simulink model "MPPT_INC"  (R2018a)
settings: Solver=ode23s  StartTime=0.0  StopTime=1200  MaxStep=1e-5  RelTol=1e-4  EnableMultiTasking=on
libraries: powerlib x7, powerlib_meascontrol x1, re_lib x1, simulink x1
settings Model: Creator=HP  LastModifiedBy=yusuf
settings SolverCC: ZeroCrossControl=DisableAll  AlgebraicLoopSolver=LineSearch
settings DataIOCC: LimitDataPoints=on  SaveFormat=Array
settings OptimizationCC: LifeSpan=inf
settings DebuggingCC: SFUnexpectedBacktrackingDiag=warning  SFNoUnconditionalDefaultTransitionDiag=warning  SFExecutionAtInitializationDiag=none
settings HardwareCC: ProdBitPerPointer=32  ProdBitPerSizeT=32  ProdBitPerPtrDiffT=32  ProdLargestAtomicFloat=None  ProdIntDivRoundTo=Undefined  ProdEndianess=Unspecified  ProdWordSize=32  ProdHWDeviceType=32-bit Generic
settings ModelReferenceCC: PropagateSignalLabelsOutOfModel=off
settings CodeAppCC: StateflowObjectComments=on
settings GRTTargetCC: TargetLangStandard=C89/C90 (ANSI)  GeneratePreprocessorConditionals=Disable all
settings ConfigComp: CovMetricSettings=dw  CovHtmlReporting=on  CovSaveCumulativeToWorkspaceVar=on  CovSaveSingleToWorkspaceVar=on  CovExternalEMLEnable=off
settings SimscapeCC: SimscapeNormalizeSystem=off

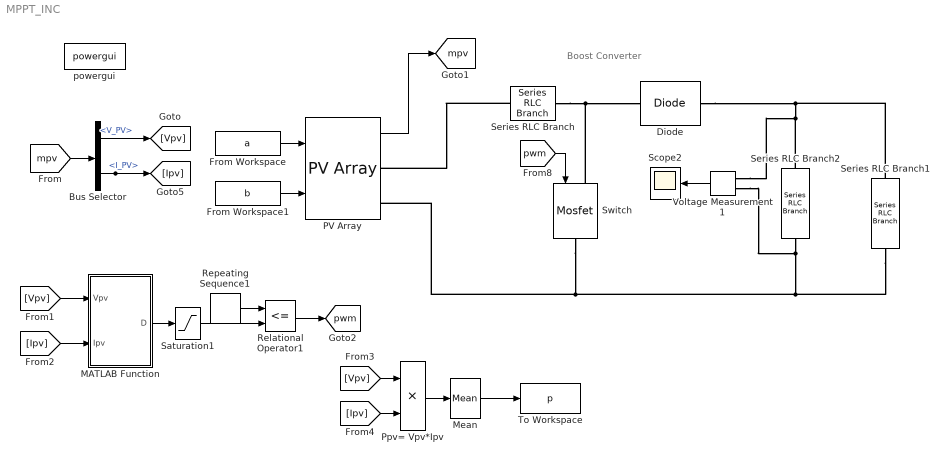
== system MPPT_INC ==
  note: Boost Converter
  Bus Selector : BusSelector  OutputSignals=V_PV,I_PV
  Diode : powerlib/Power Electronics/Diode  Ron=0.000000001  Lon=0  Vf=0  IC=0  UseSnubber=0  Rs=inf  Cs=250e-9  Measurements=off
  From Workspace : FromWorkspace  VariableName=a  SampleTime=1.5
  From Workspace1 : FromWorkspace  VariableName=b  SampleTime=1.5
  MATLAB Function : MATLAB Function  TreatAsAtomicUnit=on
  Mean : powerlib_meascontrol/Measurements/Mean  Freq=5000  Vinit=0  Ts=0
  PV Array : re_lib/Solar/PV Array  Npar=64  Nser=5  PlotType=array @ 1000 W/m2 & specified temperatures  S_vec="[ 1000  500  100 ]"  Temp_C_vec="[ 35 45 55 65 75  ]"  ModuleName=MX Solar USA MX60-220  PlotWhenSelected=on  Pm=219.929  Ncell=60  Voc=36.5  Isc=8.24  Vm=28.9  Im=7.61  beta_Voc_pc=-0.36901  alpha_Isc_pc=0.087998  beta_Voc=-0.13469  alpha_Isc=0.007251  IL=8.2621  I0=3.9406e-10  nI=0.9975  Rsh=154.3792  Rs=0.41403  BAL=off  Tc=1e-6  Tfilter=5e-5
  Ppv= Vpv*Ipv : Product
  Relational Operator1 : RelationalOperator  Operator=<=  OutDataTypeStr=boolean  ZeroCross=off  RndMeth=Nearest
  Repeating Sequence1 : simulink/Sources/Repeating Sequence  rep_seq_t="[0  1]/5000"  rep_seq_y=[0 1 ]
  Saturation1 : Saturate  UpperLimit=1  LowerLimit=0
  Scope2 : Scope
  Series RLC Branch : powerlib/Elements/Series RLC Branch  LConnTagsString=__new0  RConnTagsString=__new0  BranchType=L  Resistance=1  Inductance=5e-3  SetiL0=off  InitialCurrent=0  Capacitance=1e-6  Setx0=off  InitialVoltage=0  Measurements=None
  Series RLC Branch1 : powerlib/Elements/Series RLC Branch  LConnTagsString=__new0  RConnTagsString=__new0  BranchType=R  Resistance=50  Inductance=1e-3  SetiL0=off  InitialCurrent=0  Capacitance=9400e-6  Setx0=on  InitialVoltage=600  Measurements=None
  Series RLC Branch2 : powerlib/Elements/Series RLC Branch  LConnTagsString=__new0  RConnTagsString=__new0  BranchType=C  Resistance=1  Inductance=1e-3  SetiL0=off  InitialCurrent=0  Capacitance=100e-6  Setx0=off  InitialVoltage=600  Measurements=None
  Switch : powerlib/Power Electronics/Mosfet  Ron=0.00001  Lon=0  Rd=0.00001  Vfd=0  IC=0  Rs=1e5  Cs=inf  Measurements=off
  To Workspace : ToWorkspace  VariableName=p  SaveFormat=Timeseries  SampleTime=0.1
  Voltage Measurement1 : powerlib/Measurements/Voltage Measurement  PhasorSimulation=off  OutputType=Complex  PSBequivalent=0
  powergui : powerlib/powergui  SimulationMode=Discrete  SampleTime=1e-5  frequency=60  Iterations=50  frequencyindice=0  Pbase=100e6  ErrMax=1e-4  UnitsV=kV  UnitsW=MW  buscounter=0  FunctionMessages=off  echomessages=off  EnableUseOfTLC=off  CurrentSourceSwitches=off  DisableSnubberDevices=off  DisableRonSwitches=off  DisableVfSwitches=off  DisplayEquations=off  SolverType=Backward Euler  Interpol=off  ExternalGateDelay=off  methode=off  Ts=0  x0status=blocks  SPID=off  SwTol=0  HookPort=off  RestoreLinks=warning  ResistiveCurrentMeasurement=off  Frange=[0:2:500]  Ylog=off  Xlog=on  ShowGrid=off  save=off  variable=ZData  structure=currents  ZoomFFT=off  StartTime=0.1  cycles=5  DisplayStyle=1  fundamental=50  FreqAxis=on  MaxFrequency=1000  frequencyindicesteady=1  RmsSteady=1  display=off
  tag scope: mpv=global, pwm=global
  wires:
  From Workspace/1 -> PV Array/1
  From Workspace1/1 -> PV Array/2
  Voltage Measurement1/1 -> Scope2/1
  [pwm] -> Switch/1
  PV Array/1 -> [mpv]
  Bus Selector/2 -> [Ipv]  "<I_PV>"
  Bus Selector/1 -> [Vpv]  "<V_PV>"
  [mpv] -> Bus Selector/1
  [Vpv] -> Ppv= Vpv*Ipv/1
  [Ipv] -> Ppv= Vpv*Ipv/2
  [Ipv] -> MATLAB Function/2(Ipv)
  [Vpv] -> MATLAB Function/1(Vpv)
  MATLAB Function/1(D) -> Saturation1/1
  Relational Operator1/1 -> [pwm]
  Saturation1/1 -> Relational Operator1/2
  Mean/1 -> To Workspace/1
  Ppv= Vpv*Ipv/1 -> Mean/1
  Repeating Sequence1/1 -> Relational Operator1/1
  connections:
  Series RLC Branch2/LConn1 -- Series RLC Branch1/LConn1 -- Diode/RConn1 -- Voltage Measurement1/LConn1
  Switch/LConn1 -- Series RLC Branch/RConn1 -- Diode/LConn1
  Voltage Measurement1/LConn2 -- Series RLC Branch2/RConn1 -- Series RLC Branch1/RConn1 -- PV Array/RConn2 -- Switch/RConn1
  Series RLC Branch/LConn1 -- PV Array/RConn1

== matlab function MPPT_INC/MATLAB Function ==
  settings: updateMethod=DISCRETE
  data: Vpv input; D output; Ipv input
function D = MPPT_IC(Vpv,Ipv)

del=0.00001; 
do=0;
dmin=0;
dmax=1;

persistent Vold Dold Iold;

if isempty(Vold)
    Vold = 0;
    Iold = 0;
    Dold = do;
end
dv=Vpv - Vold;
di=Ipv - Iold;

if dv == 0
    if di == 0
        D = Dold;
    else
        if di > 0
            D = Dold - del;
        else
            D = Dold + del;
        end
    end
else
    if di/dv == -(Ipv/Vpv)
        D = Dold;
    else 
        if di/dv > -(Ipv/Vpv)
            D = Dold - del;
        else
            D = Dold + del;
        end
    end
end

Dold = D;
Vold = Vpv;
Iold = Ipv;
end
